simulink model "prova"  (R2023b)
settings: Solver=ode4  StartTime=0.0  StopTime=tf  FixedStep=t_step  RelTol=1e-3
values from neighbouring files (symbols this model uses):
  ARW = ARW*[1 1 1]'    [gyroscope.m]
  bias = bias*[1 1 1]'    [gyroscope.m]
  I = [Ix 0 0; 0 Iy 0; 0 0 Iz]    [gyroscope.m]
  I_inv = inv(I)    [gyroscope.m]
undefined symbols (not defined in the file or in its folder): A_1, A_2, A_3, A_4, A_5, A_6, alpha, DCM_eci_per, e, FS, H0, h_r_0, i, I_RW, I_vector_RW, inc_tot, InitialTrueAnomalyOfEarth, j_b, matrix_RW_config, matrix_RW_config_inv, mu_E, N_1, N_2, N_3, N_4, N_5, N_6, n_e, p, q0, r_1, r_2, r_3, r_4, r_5, r_6, R_E, rho_d1, rho_d2, rho_d3, rho_d4, rho_d5, rho_d6, rho_s1, rho_s2, rho_s3, rho_s4, rho_s5, rho_s6, t_step, th0, ts_sensor, w0, w0_RW, w_E, wMax_RW
libraries: matrix_library x28, simulink x4, dspindex x3, vrlib x2, aerolibutil x1
(part 1 of 2)
settings Model: Creator=samue  LastModifiedBy=samue

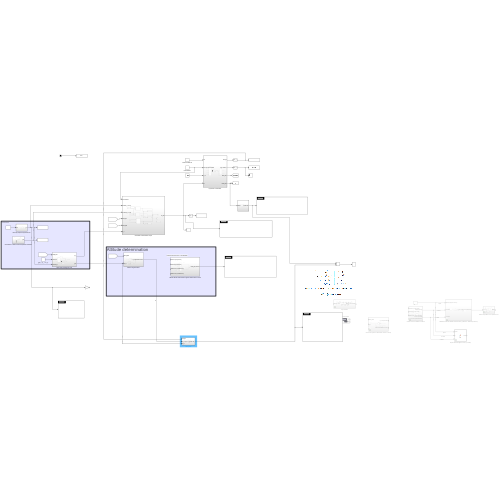
[thumbnail: Simulink's stored preview of the top-level diagram]
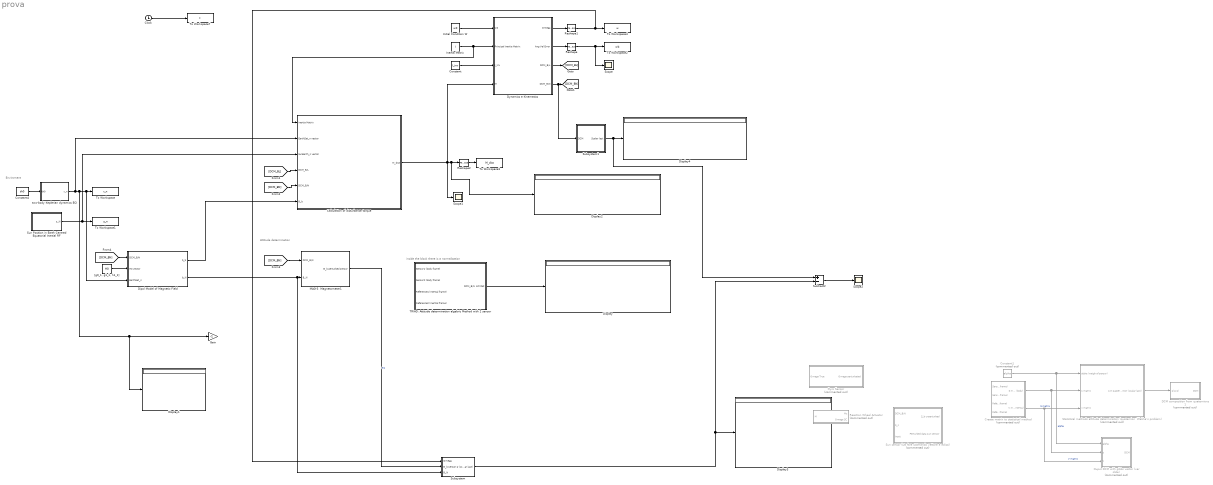
== system prova ==
  note: Attitude determination
  note: inside the block there is a normalisation
  note: Enviroment
  Calculation of disturbance torque : Subsystem
  Clock : Clock
  Constant : Constant  Value=I_inv
  Constant1 : Constant  Commented=on  Value=alpha
  Constant4 : Constant  Value=th0
  Create matrix to statistical method : Subsystem  Commented=on
  DCM composition from quaternions 1 : Subsystem  Commented=on  AncestorBlock=LibrarySAD5/DCM composition from quaternions
  Dipol Model of Magnetic Field : Subsystem
  Display{,1..4} (5 alike) : Display
  Dynamics e Kinematics : Subsystem
  Gain : Gain  Gain=-1
  Gyro Sensor : Subsystem  Commented=on
  Inertia Matrix : Constant  Value=I  VectorParams1D=off
  Initial Condition W : Constant  Value=w0
  MAG-3  Magnetometer1 : Subsystem
  Ouput DCM with gibbs vector (ver slide) : MATLAB Function  Commented=on  TreatAsAtomicUnit=on
  Reaction Wheel Actuator : Subsystem  Commented=on
  Reshape : Reshape
  Reshape1 : Reshape
  Reshape2 : Reshape
  Scope : Scope
  Scope1 : Scope
  Scope2 : Scope
  "Statistical methods attitude determination (quaternion  Wabha’s problem) " : Subsystem  Commented=on
  Subsystem : Subsystem
  Subsystem1 : Subsystem
  Subtract2 : Sum  Inputs=+-
  Sun Position in Earth Centred Equatorial Inertial RF : Subsystem
  Sun sensor (Da fare sistmando vettore e eclissi) : Subsystem  Commented=on
  TRIAD: Attitude determination algebric Method with 2 sensor : Subsystem
  To Workspace : ToWorkspace  VariableName=r_n  SampleTime=-1
  To Workspace1 : ToWorkspace  VariableName=s_n  SampleTime=-1
  To Workspace2 : ToWorkspace  VariableName=wb  SampleTime=-1
  To Workspace3 : ToWorkspace  VariableName=M_dist  SaveFormat=Timeseries  SampleTime=-1
  To Workspace4 : ToWorkspace  VariableName=w  SampleTime=-1
  To Workspace7 : ToWorkspace  VariableName=t  SampleTime=-1
  "[g0_1, g1_1, h1_1]" : Constant  Value=H0
  two-body Keplerian dynamics ECI : Subsystem
  wires:
  Inertia Matrix/1 -> Calculation of disturbance torque/1(Inertia Matrix), Dynamics e Kinematics/2(Principal Inertia Matrix)
  [DCM_BN] -> MAG-3  Magnetometer1/1(DCM_B/N)
  Constant4/1 -> two-body Keplerian dynamics ECI/1(th0)
  Constant/1 -> Dynamics e Kinematics/3(I_inv)
  [DCM_BL] -> Calculation of disturbance torque/4(DCM_B/L)
  Sun Position in Earth Centred Equatorial Inertial RF/1(s_N) -> To Workspace1/1, Calculation of disturbance torque/3(SunEarth_n vector)
  Reshape1/1 -> Subsystem/1(Omega), To Workspace4/1
  Dynamics e Kinematics/3(DCM_B/L) -> [DCM_BL]
  Reshape/1 -> Scope/1, To Workspace2/1
  Calculation of disturbance torque/1(M_dist) -> Display2/1, Reshape2/1, Dynamics e Kinematics/4(M), Scope1/1
  Dynamics e Kinematics/2(Ang Vel Error) -> Reshape/1
  Reshape2/1 -> To Workspace3/1
  "[g0_1, g1_1, h1_1]"/1 -> Dipol Model of Magnetic Field/2(H0 vector)
  "Statistical methods attitude determination (quaternion  Wabha’s problem) "/1(q in quaternion (scalar last)) -> DCM composition from quaternions 1/1(q(4x1))
  Dynamics e Kinematics/1(Omega) -> Reshape1/1
  Dynamics e Kinematics/4(DCM_B/N) -> Subsystem1/1(DCM), [DCM_BN]
  Clock/1 -> To Workspace7/1
  [DCM_BN] -> Dipol Model of Magnetic Field/1(DCM_B/N)
  Dipol Model of Magnetic Field/1(b_b) -> Calculation of disturbance torque/6(B_b)
  Create matrix to statistical method/2(V matrix (inertia)) -> "Statistical methods attitude determination (quaternion  Wabha’s problem) "/3(v matrix), Ouput DCM with gibbs vector (ver slide)/3(v)  "V matrix"
  Initial Condition W/1 -> Dynamics e Kinematics/1(w0)
  [DCM_BN] -> Calculation of disturbance torque/5(DCM_B/N)
  TRIAD: Attitude determination algebric Method with 2 sensor/1(DCM_B/N  Att Det) -> Display/1
  two-body Keplerian dynamics ECI/1(r_n) -> Calculation of disturbance torque/2(EarthSat_n vector), To Workspace/1, Dipol Model of Magnetic Field/3(EarthSat_n), Display1/1, Gain/1
  Create matrix to statistical method/1(S matrix (body)) -> "Statistical methods attitude determination (quaternion  Wabha’s problem) "/2(s matrix), Ouput DCM with gibbs vector (ver slide)/2(s)  "S matrix"
  Constant1/1 -> "Statistical methods attitude determination (quaternion  Wabha’s problem) "/1(alpha (weigh of sensor)), Ouput DCM with gibbs vector (ver slide)/1(alpha)  "alpha"
  Dipol Model of Magnetic Field/2(b_N) -> Subsystem/3(B_N), MAG-3  Magnetometer1/2(B_N)
  Subsystem1/1(Scalar last) -> Subtract2/1, Display4/1
  Subtract2/1 -> Scope2/1
  Subsystem/1(q (scalar last)) -> Subtract2/2, Display3/1
  MAG-3  Magnetometer1/1(B_b perturbed sensor) -> Subsystem/2(B_b sensor)  "B1"

== system prova/Calculation of disturbance torque ==
  Inertia Matrix : Inport
  EarthSat_n vector : Inport  Port=2
  SunEarth_n vector : Inport  Port=3
  DCM_B/L : Inport  Port=4
  DCM_B/N : Inport  Port=5
  B_b : Inport  Port=6
  Display : Display
  Extract Diagonal : matrix_library/Extract Diagonal
      settings: LibrarySourceBlock=|
      | simulink/Matrix
      | Operations/Extract Diagonal
  M of gravity gradient1 : Subsystem
  Magnetic Torque : Subsystem
  Reshape : Reshape
  Reshape1 : Reshape
  Scope : Scope
  Solar pressure on 6 faces : Subsystem  Commented=on
  Sum : Sum  Inputs=|+++
  Terminator : Terminator  Commented=on
  To Workspace1 : ToWorkspace  VariableName=M_b  SampleTime=-1
  To Workspace3 : ToWorkspace  VariableName=M_GG  SampleTime=-1
  To Workspace8 : ToWorkspace  VariableName=M_SRP  SampleTime=-1
  j_b : Constant  Value=j_b
  M_dist : Outport
  wires:
  DCM_B/L/1 -> M of gravity gradient1/2(A_B/L)
  j_b/1 -> Magnetic Torque/1(j_b)
  Magnetic Torque/1(M_b) -> Sum/3, Reshape1/1
  B_b/1 -> Magnetic Torque/2(B_b)
  Inertia Matrix/1 -> Extract Diagonal/1
  EarthSat_n vector/1 -> M of gravity gradient1/3(r_N), Solar pressure on 6 faces/2(S_N)
  DCM_B/N/1 -> Solar pressure on 6 faces/1(DCM)
  SunEarth_n vector/1 -> Solar pressure on 6 faces/3("r_N ")
  Sum/1 -> M_dist/1
  Reshape/1 -> To Workspace8/1
  Reshape1/1 -> To Workspace1/1
  M of gravity gradient1/1(GravityGradient_M) -> Reshape/1, To Workspace3/1, Sum/1
  Solar pressure on 6 faces/2(Ftot_SP) -> Terminator/1
  Solar pressure on 6 faces/1(Mtot_SP) -> Display/1, Scope/1, Sum/2
  Extract Diagonal/1 -> M of gravity gradient1/1(Inertia Vector)

== system prova/Create matrix to statistical method ==
  Sensor1 (body frame) : Inport
  Sensor2 (body frame) : Inport  Port=2
  Reference1 (Inertial frame) : Inport  Port=3
  Reference2 (Inertial frame) : Inport  Port=4
  Matrix Concatenate1 : Concatenate  Mode=Multidimensional array  ConcatenateDimension=2
  Matrix Concatenate2 : Concatenate  Mode=Multidimensional array  ConcatenateDimension=2
  Normalize Vector1 : Subsystem
  Normalize Vector2 : Subsystem
  Normalize Vector3 : Subsystem
  Normalize Vector4 : Subsystem
  S matrix (body) : Outport
  V matrix (inertia) : Outport  Port=2
  wires:
  Matrix Concatenate1/1 -> V matrix (inertia)/1
  Normalize Vector1/1(Versor) -> Matrix Concatenate2/1
  Normalize Vector2/1(Versor) -> Matrix Concatenate2/2
  Normalize Vector4/1(Versor) -> Matrix Concatenate1/2
  Normalize Vector3/1(Versor) -> Matrix Concatenate1/1
  Matrix Concatenate2/1 -> S matrix (body)/1
  Reference1 (Inertial frame)/1 -> Normalize Vector3/1(Vector)
  Reference2 (Inertial frame)/1 -> Normalize Vector4/1(Vector)
  Sensor1 (body frame)/1 -> Normalize Vector1/1(Vector)
  Sensor2 (body frame)/1 -> Normalize Vector2/1(Vector)

== system prova/DCM composition from quaternions 1 ==
  q(4x1) : Inport
  Cross product matrix composition : Subsystem
  Demux : Demux
  Dot Product : DotProduct  OutDataTypeStr=Inherit: Inherit via internal rule
  Gain : Gain  Gain=[1 0 0; 0 1 0; 0 0 1]
  Gain1 : Gain  Gain=2
  Gain2 : Gain  Gain=-2
  Mux : Mux  Inputs=3
  Product : Product  Multiplication=Matrix(*)
  Product1 : Product
  Square : Math  Operator=square
  Sum : Sum  Inputs=|-+
  Sum1 : Sum  Inputs=+++
  Transpose : Math  Operator=transpose
  DCM : Outport
  wires:
  Gain/1 -> Sum1/1
  Demux/1 -> Mux/1
  q(4x1)/1 -> Demux/1
  Demux/2 -> Mux/2
  Mux/1 -> Dot Product/2, Dot Product/1, Product/1, Cross product matrix composition/1(q_vect), Transpose/1  "q_vect"
  Demux/4 -> Gain2/1, Square/1  "q4"
  Demux/3 -> Mux/3
  Dot Product/1 -> Sum/1
  Sum/1 -> Gain/1
  Square/1 -> Sum/2
  Transpose/1 -> Product/2
  Product/1 -> Gain1/1
  Gain2/1 -> Product1/2
  Cross product matrix composition/1(q_vect cross) -> Product1/1  "omega_mat"
  Product1/1 -> Sum1/3
  Gain1/1 -> Sum1/2
  Sum1/1 -> DCM/1

== system prova/Dipol Model of Magnetic Field ==
  note: CODE TO ADD
      | % Definition of Magnetic Field (Dipole model)
      |  j_b = [0.01 0.05 0.01]';
      | H0 = 1e-9.*[-29404.8 -1450.9 4652.5]';
  DCM_B/N : Inport
  H0 vector : Inport  Port=2
  EarthSat_n : Inport  Port=3
  Calculation of b_n : Subsystem
  Matrix Multiply : Product  Multiplication=Matrix(*)
  To Workspace : ToWorkspace  VariableName=bn  SampleTime=-1
  b_b : Outport
  b_N : Outport  Port=2
  wires:
  Matrix Multiply/1 -> b_b/1
  DCM_B/N/1 -> Matrix Multiply/1
  H0 vector/1 -> Calculation of b_n/1(H0 vector)
  EarthSat_n/1 -> Calculation of b_n/2(EarthSat_n)
  Calculation of b_n/1(b_N) -> Matrix Multiply/2, To Workspace/1, b_N/1

== system prova/Dynamics e Kinematics ==
  w0 : Inport
  Principal Inertia Matrix : Inport  Port=2
  I_inv : Inport  Port=3
  M : Inport  Port=4
  Attitude error GG : Subsystem
  Constant6 : Constant  Value=q0
  DCM composition from quaternions 1 : Subsystem  AncestorBlock=LibrarySAD5/DCM composition from quaternions
  Kinematics quaternion2 : Subsystem
  Single spin dynamics : Subsystem  AncestorBlock=My_library/Single spin dynamics
  Terminator1 : Terminator
  Omega : Outport
  Ang Vel Error : Outport  Port=2
  DCM_B/L : Outport  Port=3
  DCM_B/N : Outport  Port=4
  wires:
  DCM composition from quaternions 1/1(DCM) -> DCM_B/N/1, Attitude error GG/2(DCM_B/N)
  Constant6/1 -> Kinematics quaternion2/2(q0)
  Single spin dynamics/1(Omega) -> Omega/1, Attitude error GG/1(w), Kinematics quaternion2/1(omega)
  Kinematics quaternion2/2(q^(-1)) -> Terminator1/1
  M/1 -> Single spin dynamics/4(M)
  w0/1 -> Single spin dynamics/3(Omega_0)
  Principal Inertia Matrix/1 -> Single spin dynamics/2(Inertia matrix)
  Kinematics quaternion2/1(q) -> DCM composition from quaternions 1/1(q(4x1))
  Attitude error GG/2(DCM_B/L) -> DCM_B/L/1
  Attitude error GG/1(Ang Vel Error) -> Ang Vel Error/1
  I_inv/1 -> Single spin dynamics/1(Inertia matrix inverse)

== system prova/Gyro Sensor ==
  Omega True : Inport
  Band-Limited White Noise : simulink/Sources/Band-Limited White Noise  Cov=[0.00001]  Ts=0.1  seed=[23341]
  Constant : Constant  Value=ARW  VectorParams1D=off
  Constant1 : Constant  Value=bias  VectorParams1D=off
  Sum : Sum  Inputs=|++
  Sum1 : Sum  Inputs=|++
  Sum2 : Sum  Inputs=|++
  Zero-Order Hold : ZeroOrderHold  SampleTime=-1
  Omega perturbated : Outport
  wires:
  Zero-Order Hold/1 -> Sum/1
  Sum2/1 -> Omega perturbated/1
  Sum1/1 -> Sum2/1
  Sum/1 -> Sum1/1
  Omega True/1 -> Zero-Order Hold/1
  Constant1/1 -> Sum2/2
  Band-Limited White Noise/1 -> Sum/2
  Constant/1 -> Sum1/2

== system prova/MAG-3  Magnetometer1 ==
  note: CODE TO ADD TO MAKE SENSOR WORK
      | % Time definition
      | t0 = 0;
      | tf = T; %Period of orbit
      | t_step = 0.01; %fixed step of simulation
      | ts_sensor = t_step; % Sample of sensor (can change but must to be a multiple of t_step)
      |
      | % MAG-3 sensor data and error
      | FS = 500e-9; %Full scale value
      | inc_lin = 0.15/100; % Accuracy error
      | inc_acc = 0.75/100; % Linear error
      | inc_tot = sqrt(inc_lin^2 + inc_acc^2); %Total error
  DCM_B/N : Inport
  B_N : Inport  Port=2
  Error gain of sensor MAG-3 : Gain  Gain=inc_tot*FS
  Rotation in body frame : Product  Multiplication=Matrix(*)
  Saturation to FS : Saturate  UpperLimit=FS  LowerLimit=-FS
  Sum : Sum  Inputs=|++
  Vector Concatenate : Concatenate  NumInputs=3
  White Noise : RandomNumber  DisableCoverage=on  Seed=1  SampleTime=ts_sensor
  White Noise1 : RandomNumber  DisableCoverage=on  Seed=2  SampleTime=ts_sensor
  White Noise2 : RandomNumber  DisableCoverage=on  Seed=3  SampleTime=ts_sensor
  Zero-Order Hold : ZeroOrderHold  SampleTime=ts_sensor
  B_b perturbed sensor : Outport
  wires:
  Vector Concatenate/1 -> Error gain of sensor MAG-3/1
  White Noise/1 -> Vector Concatenate/1
  Error gain of sensor MAG-3/1 -> Sum/2
  White Noise2/1 -> Vector Concatenate/3
  White Noise1/1 -> Vector Concatenate/2
  DCM_B/N/1 -> Rotation in body frame/1
  B_N/1 -> Zero-Order Hold/1
  Zero-Order Hold/1 -> Rotation in body frame/2
  Saturation to FS/1 -> B_b perturbed sensor/1
  Rotation in body frame/1 -> Sum/1
  Sum/1 -> Saturation to FS/1

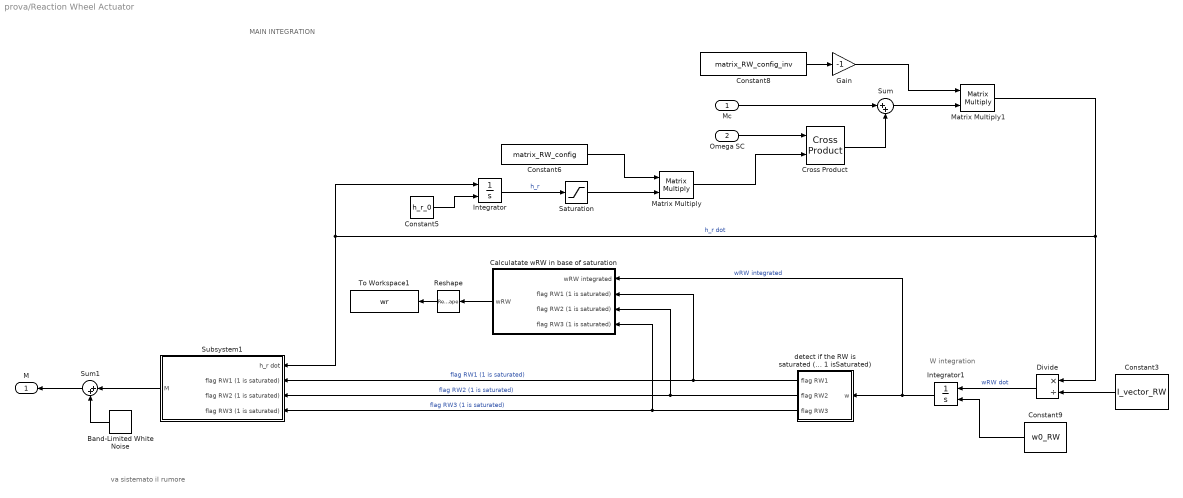
== system prova/Reaction Wheel Actuator ==
  note: W integration
  note: va sistemato il rumore
  note: MAIN INTEGRATION
  Mc : Inport
  Omega SC : Inport  Port=2
  Band-Limited White Noise : simulink/Sources/Band-Limited White Noise  Cov=[0.00001]  Ts=t_step  seed=[23341]
  Calculatate wRW in base of saturation : Subsystem
  Constant3 : Constant  Value=I_vector_RW
  Constant5 : Constant  Value=h_r_0  VectorParams1D=off
  Constant6 : Constant  Value=matrix_RW_config  VectorParams1D=off
  Constant8 : Constant  Value=matrix_RW_config_inv  VectorParams1D=off
  Constant9 : Constant  Value=w0_RW
  Cross Product : matrix_library/Cross Product
  Divide : Product  Inputs=*/
  Gain : Gain  Gain=-1
  Integrator : Integrator  InitialConditionSource=external
  Integrator1 : Integrator  InitialConditionSource=external
  Matrix Multiply : Product  Multiplication=Matrix(*)
  Matrix Multiply1 : Product  Multiplication=Matrix(*)
  Reshape : Reshape
  Saturation : Saturate  UpperLimit=wMax_RW*I_RW  LowerLimit=-wMax_RW*I_RW
  Subsystem1 : Subsystem
  Sum : Sum  Inputs=|++
  Sum1 : Sum  Inputs=|++
  To Workspace1 : ToWorkspace  VariableName=wr  SampleTime=-1
  detect if the RW is saturated (output == 1 isSaturated) : Subsystem
  M : Outport
  wires:
  Matrix Multiply1/1 -> Integrator/1, Subsystem1/1(h_r dot), Divide/1  "h_r dot"
  Constant6/1 -> Matrix Multiply/1
  Cross Product/1 -> Sum/2
  Constant8/1 -> Gain/1
  Sum/1 -> Matrix Multiply1/2
  detect if the RW is saturated (output == 1 isSaturated)/2(flag RW2) -> Calculatate wRW in base of saturation/3(flag RW2 (1 is saturated)), Subsystem1/3(flag RW2 (1 is saturated))  "flag RW2 (1 is saturated)"
  Calculatate wRW in base of saturation/1(wRW) -> Reshape/1
  Matrix Multiply/1 -> Cross Product/2
  Constant5/1 -> Integrator/2
  Constant3/1 -> Divide/2
  Gain/1 -> Matrix Multiply1/1
  Mc/1 -> Sum/1
  Saturation/1 -> Matrix Multiply/2
  Integrator1/1 -> Calculatate wRW in base of saturation/1(wRW integrated), detect if the RW is saturated (output == 1 isSaturated)/1(w)  "wRW integrated"
  Constant9/1 -> Integrator1/2
  Divide/1 -> Integrator1/1  "wRW dot"
  Integrator/1 -> Saturation/1  "h_r"
  detect if the RW is saturated (output == 1 isSaturated)/3(flag RW3) -> Calculatate wRW in base of saturation/4(flag RW3 (1 is saturated)), Subsystem1/4(flag RW3 (1 is saturated))  "flag RW3 (1 is saturated)"
  detect if the RW is saturated (output == 1 isSaturated)/1(flag RW1) -> Calculatate wRW in base of saturation/2(flag RW1 (1 is saturated)), Subsystem1/2(flag RW1 (1 is saturated))  "flag RW1 (1 is saturated)"
  Reshape/1 -> To Workspace1/1
  Omega SC/1 -> Cross Product/1
  Subsystem1/1(M) -> Sum1/1
  Sum1/1 -> M/1
  Band-Limited White Noise/1 -> Sum1/2

== system prova/Statistical methods attitude determination (quaternion  Wabha’s problem)  ==
  note: In questo blocco ci sono altri metodi per il calcolo di q
  note: BLOCCO DA SISTEMARE SCEGLIENDO UNA SOLUZIONE
  note: Resolve linear system:
      | (𝑆 − σI)𝑞 + zq_4 = 𝜆_(MAX)*𝑞
      | 𝑧'𝑞 + σ*q_4 = 𝜆_(MAX)*𝑞_4
      |
      | Calculate eigenvalue (in the theory we assumed that lambda_max = 1)
  note: 𝐾 = [ (𝑆 − σI), 𝑧
      | 𝑧 ' 𝜎 ]
  note: 𝑧 = [𝑏23 − 𝑏32 , b31 − 𝑏13 , b12 − 𝑏21] '
  alpha (weigh of sensor) : Inport
  s matrix : Inport  Port=2
  v matrix : Inport  Port=3
  Adjoint of 3x3 Matrix : aerolibutil/Adjoint of 3x3 Matrix
  Blocco da convertire in formato simulink. Ho trovato 3 soluzioni differenti al proble : MATLAB Function  TreatAsAtomicUnit=on
  For Iterator Subsystem to calculate B matrix : Subsystem  TreatAsAtomicUnit=on
  Gain : Gain  Gain=eye(3)
  Matrix Concatenate : Concatenate  Mode=Multidimensional array  ConcatenateDimension=2
  Matrix Concatenate1 : Concatenate  Mode=Multidimensional array
  Matrix trace : Subsystem
  Subtract : Sum  Inputs=+-
  Sum : Sum  Inputs=|++
  Transpose : Math  Operator=transpose
  Transpose2 : Math  Operator=transpose
  Vector Concatenate1 : Concatenate
  Vector z : Subsystem
  q in quaternion (scalar last) : Outport
  wires:
  Transpose/1 -> Sum/2
  For Iterator Subsystem to calculate B matrix/1(B matrix) -> Vector z/1(B), Matrix trace/1(Matrix), Transpose/1, Sum/1  "B matrix"
  Sum/1 -> Adjoint of 3x3 Matrix/1, Blocco da convertire in formato simulink. Ho trovato 3 soluzioni differenti al proble/2(S), Subtract/1  "matrix S"
  Gain/1 -> Subtract/2
  Matrix trace/1(trace) -> Vector Concatenate1/2, Gain/1  "sigma = tr(B)"
  Matrix Concatenate/1 -> Matrix Concatenate1/1
  Vector Concatenate1/1 -> Transpose2/1
  Vector z/1(z) -> Vector Concatenate1/1, Matrix Concatenate/2
  Transpose2/1 -> Matrix Concatenate1/2
  Subtract/1 -> Matrix Concatenate/1  "S - sigma*eye(3)"
  alpha (weigh of sensor)/1 -> For Iterator Subsystem to calculate B matrix/1(alpha)
  v matrix/1 -> For Iterator Subsystem to calculate B matrix/3(v matrix)
  s matrix/1 -> For Iterator Subsystem to calculate B matrix/2(s matrix)
  Blocco da convertire in formato simulink. Ho trovato 3 soluzioni differenti al proble/1(q) -> q in quaternion (scalar last)/1  "q in quaternion (scalar last)"
  Adjoint of 3x3 Matrix/1 -> Blocco da convertire in formato simulink. Ho trovato 3 soluzioni differenti al proble/3(Sadj)
  Matrix Concatenate1/1 -> Blocco da convertire in formato simulink. Ho trovato 3 soluzioni differenti al proble/1(K)  "K matrix"

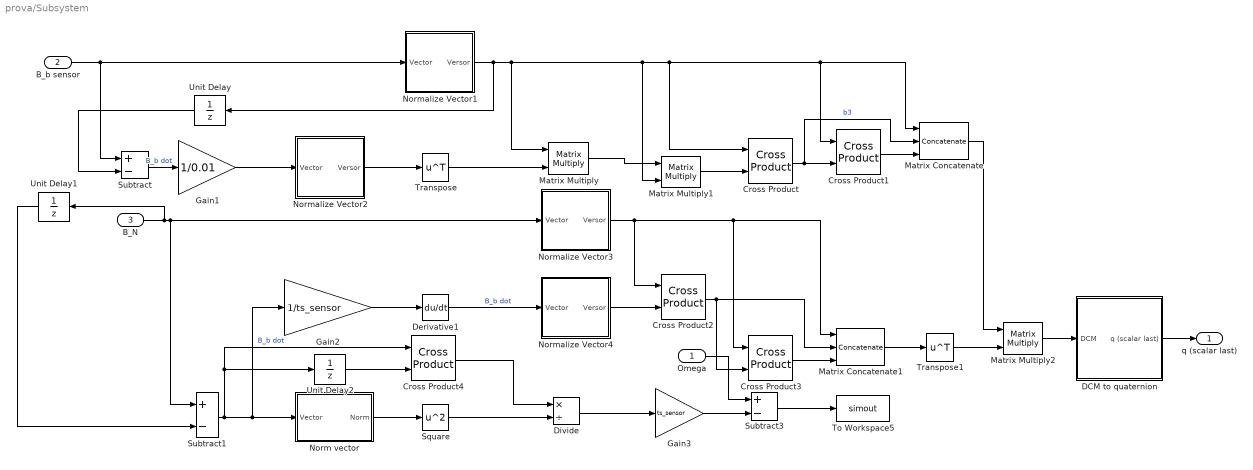
== system prova/Subsystem ==
  Omega : Inport
  B_b sensor : Inport  Port=2
  B_N : Inport  Port=3
  Cross Product{,1..4} (5 alike) : matrix_library/Cross Product
  DCM to quaternion : Subsystem
  Derivative1 : Derivative
  Divide : Product  Inputs=*/
  Gain1 : Gain  Gain=1/0.01
  Gain2 : Gain  Gain=1/ts_sensor
  Gain3 : Gain  Gain=ts_sensor
  Matrix Concatenate : Concatenate  NumInputs=3  Mode=Multidimensional array  ConcatenateDimension=2
  Matrix Concatenate1 : Concatenate  NumInputs=3  Mode=Multidimensional array  ConcatenateDimension=2
  Matrix Multiply : Product  Multiplication=Matrix(*)
  Matrix Multiply1 : Product  Multiplication=Matrix(*)
  Matrix Multiply2 : Product  Multiplication=Matrix(*)
  Norm vector : Subsystem  AncestorBlock=LibrarySAD5/Normalize Vector1
  Normalize Vector1 : Subsystem
  Normalize Vector2 : Subsystem
  Normalize Vector3 : Subsystem
  Normalize Vector4 : Subsystem
  Square : Math  Operator=square
  Subtract : Sum  Inputs=+-
  Subtract1 : Sum  Inputs=+-
  Subtract3 : Sum  Inputs=+-
  To Workspace5 : ToWorkspace  VariableName=simout  SaveFormat=Timeseries  SampleTime=-1
  Transpose : Math  Operator=transpose
  Transpose1 : Math  Operator=transpose
  Unit Delay : UnitDelay  SampleTime=-1  HasFrameUpgradeWarning=on
  Unit Delay1 : UnitDelay  SampleTime=-1  HasFrameUpgradeWarning=on
  Unit Delay2 : UnitDelay  SampleTime=-1  HasFrameUpgradeWarning=on
  q (scalar last) : Outport
  wires:
  Unit Delay1/1 -> Subtract1/2
  B_b sensor/1 -> Normalize Vector1/1(Vector), Subtract/1
  Gain1/1 -> Normalize Vector2/1(Vector)
  Subtract/1 -> Gain1/1  "B_b dot"
  Unit Delay/1 -> Subtract/2
  B_N/1 -> Normalize Vector3/1(Vector), Subtract1/1, Unit Delay1/1
  Subtract1/1 -> Norm vector/1(Vector), Gain2/1, Cross Product4/1, Unit Delay2/1  "B_b dot"
  Normalize Vector2/1(Versor) -> Transpose/1
  Gain2/1 -> Derivative1/1
  Unit Delay2/1 -> Cross Product4/2
  Norm vector/1(Norm) -> Square/1
  Normalize Vector1/1(Versor) -> Cross Product1/1, Matrix Concatenate/1, Cross Product/1, Matrix Multiply1/2, Matrix Multiply/1, Unit Delay/1
  Transpose/1 -> Matrix Multiply/2
  Derivative1/1 -> Normalize Vector4/1(Vector)  "B_b dot"
  Cross Product4/1 -> Divide/1
  Square/1 -> Divide/2
  Matrix Multiply/1 -> Matrix Multiply1/1
  Normalize Vector3/1(Versor) -> Matrix Concatenate1/1, Cross Product3/1, Cross Product2/1
  Normalize Vector4/1(Versor) -> Cross Product2/2
  Divide/1 -> Gain3/1
  Matrix Multiply1/1 -> Cross Product/2
  Cross Product2/1 -> Matrix Concatenate1/2, Cross Product3/2
  Omega/1 -> Subtract3/1
  Gain3/1 -> Subtract3/2
  Cross Product/1 -> Cross Product1/2, Matrix Concatenate/2  "b3"
  Cross Product3/1 -> Matrix Concatenate1/3
  Subtract3/1 -> To Workspace5/1
  Cross Product1/1 -> Matrix Concatenate/3
  Matrix Concatenate1/1 -> Transpose1/1
  Matrix Concatenate/1 -> Matrix Multiply2/1
  Transpose1/1 -> Matrix Multiply2/2
  Matrix Multiply2/1 -> DCM to quaternion/1(DCM)
  DCM to quaternion/1(q (scalar last)) -> q (scalar last)/1

== system prova/Subsystem1 ==
  DCM : Inport
  Constant : Constant
  Divide : Product  Inputs=*/
  Extract Diagonal : matrix_library/Extract Diagonal
      settings: LibrarySourceBlock=|
      | simulink/Matrix
      | Operations/Extract Diagonal
  Gain : Gain  Gain=0.5
  Gain1 : Gain  Gain=[0 0 0; 0 0 1; 0 -1 0]
  Gain2 : Gain  Gain=[0 0 -1; 0 0 0; 1 0 0]
  Gain3 : Gain  Gain=[0 1 0; -1 0 0; 0 0 0]
  Gain4 : Gain  Gain=4
  Normalize Vector1 : Subsystem
  Sqrt : Sqrt
  Sum : Sum  Inputs=|++
  Sum of Elements{,1..3} (4 alike) : Sum  Inputs=+
  Vector Concatenate : Concatenate  NumInputs=3
  Vector Concatenate1 : Concatenate
  Scalar last : Outport
  wires:
  Extract Diagonal/1 -> Sum of Elements/1
  Sum of Elements/1 -> Sum/1
  Constant/1 -> Sum/2
  Sum/1 -> Sqrt/1
  Sqrt/1 -> Gain/1
  DCM/1 -> Gain1/1, Gain2/1, Gain3/1, Extract Diagonal/1
  Gain2/1 -> Sum of Elements1/1
  Sum of Elements1/1 -> Vector Concatenate/2
  Gain1/1 -> Sum of Elements2/1
  Sum of Elements2/1 -> Vector Concatenate/1
  Sum of Elements3/1 -> Vector Concatenate/3
  Gain3/1 -> Sum of Elements3/1
  Vector Concatenate/1 -> Divide/1
  Gain/1 -> Vector Concatenate1/2, Gain4/1
  Gain4/1 -> Divide/2
  Divide/1 -> Vector Concatenate1/1
  Vector Concatenate1/1 -> Normalize Vector1/1(Vector)
  Normalize Vector1/1(Versor) -> Scalar last/1

== system prova/Sun Position in Earth Centred Equatorial Inertial RF ==
  note: pointing Sun from Earth
      |
      | x=vernal line
      | y=perpendicular
      | z=cnp
  Clock : Clock
  Gain : Gain  Gain=cos(23.45/360*2*pi)
  Gain1 : Gain  Gain=sin(23.45/360*2*pi)
  InitialTrueAnomalyOfEarth : Constant  Value=InitialTrueAnomalyOfEarth
  MatrixMultiply : Product
  Mux : Mux  Inputs=3
  Product : Product
  Sum : Sum  Inputs=|++
  Trigonometric Function : Trigonometry  Operator=cos
  Trigonometric Function1 : Trigonometry
  mean ang vel : Constant  Value=2*pi/31536000
  mean distance : Constant  Value=149597870
  s_N : Outport
  wires:
  Trigonometric Function/1 -> Mux/1
  Gain1/1 -> Mux/3
  Mux/1 -> MatrixMultiply/2
  MatrixMultiply/1 -> s_N/1  "s_N"
  mean distance/1 -> MatrixMultiply/1
  Gain/1 -> Mux/2
  Trigonometric Function1/1 -> Gain1/1, Gain/1
  mean ang vel/1 -> Product/2
  Clock/1 -> Product/1
  InitialTrueAnomalyOfEarth/1 -> Sum/2
  Product/1 -> Sum/1
  Sum/1 -> Trigonometric Function1/1, Trigonometric Function/1

== system prova/Sun sensor (Da fare sistmando vettore e eclissi) ==
  note: SUN SENSOR DA RIFINIRE, ma Utilizzabile
      | -> Modellare non rilevamento sole (esempio eclissi)
      | -> Modellare albedo terra/luna per riflessi
      | -> Sistemare distrubi basandosi su sensore reale
  DCM_B/N : Inport
  S_n : Inport  Port=2
  Input : Inport  Port=3
  Band-Limited White Noise : simulink/Sources/Band-Limited White Noise  Cov=5e9*[1 1 1]  Ts=ts_sensor  seed=[23341]
  Normalize Vector1 : Subsystem
  Rotation in body frame : Product  Multiplication=Matrix(*)
  Rotation in body frame1 : Product  Multiplication=Matrix(*)
  Sum : Sum  Inputs=|++
  Zero-Order Hold : ZeroOrderHold  SampleTime=ts_sensor
  S_b unperturbed : Outport
  Perturbed data sun sensor : Outport  Port=2
  wires:
  Band-Limited White Noise/1 -> Sum/2
  DCM_B/N/1 -> Rotation in body frame/1, Rotation in body frame1/1
  S_n/1 -> Zero-Order Hold/1, Normalize Vector1/1(Vector)
  Normalize Vector1/1(Versor) -> Rotation in body frame/2
  Zero-Order Hold/1 -> Rotation in body frame1/2
  Rotation in body frame1/1 -> Sum/1
  Rotation in body frame/1 -> S_b unperturbed/1
  Sum/1 -> Perturbed data sun sensor/1

== system prova/TRIAD: Attitude determination algebric Method with 2 sensor ==
  note: 𝑉^(-1) = 𝑉';
      | 𝐴 = 𝑆𝑉^(-1) = 𝑆𝑉'
  note: 𝑣1 = 𝑎;
      | 𝑣2 = (𝑎 ∧ 𝑏)/|𝑎 ∧ 𝑏|;
      | 𝑣3 = 𝑎 ∧ 𝑣2
  note: S1 = 𝑝;
      | 𝑠2 = (𝑝 ∧ 𝑞)/(|𝑝 ∧ 𝑞|);
      | 𝑠3 = 𝑝 ∧ 𝑠2
  Sensor1 (body frame) : Inport
  Sensor2 (body frame) : Inport  Port=2
  Reference1 (Inertial frame) : Inport  Port=3
  Reference2 (Inertial frame) : Inport  Port=4
  Matrix Multiply : Product  Multiplication=Matrix(*)
  Normalize Vector1 : Subsystem
  Normalize Vector2 : Subsystem
  Normalize Vector3 : Subsystem
  Normalize Vector4 : Subsystem
  Subsystem : Subsystem
  Subsystem1 : Subsystem
  Transpose : Math  Operator=transpose
  DCM_B/N  Att Det : Outport
  wires:
  Sensor1 (body frame)/1 -> Normalize Vector2/1(Vector)  "q"
  Sensor2 (body frame)/1 -> Normalize Vector3/1(Vector)  "p"
  Subsystem/1("Matrix S Measurements ") -> Matrix Multiply/1  "Matrix S Measurements (body frame)"
  Normalize Vector2/1(Versor) -> Subsystem/1(versor p (body frame))
  Normalize Vector3/1(Versor) -> Subsystem/2(versor q (body frame))
  Normalize Vector1/1(Versor) -> Subsystem1/1(versor a (body frame))
  Reference2 (Inertial frame)/1 -> Normalize Vector4/1(Vector)  "b"
  Reference1 (Inertial frame)/1 -> Normalize Vector1/1(Vector)  "a"
  Subsystem1/1("Matrix V certain model ") -> Transpose/1  "Matrix V (inertial frame)"
  Normalize Vector4/1(Versor) -> Subsystem1/2(versor b (body frame))
  Matrix Multiply/1 -> DCM_B/N  Att Det/1  "DCM_B/N from attirude determination"
  Transpose/1 -> Matrix Multiply/2

== system prova/two-body Keplerian dynamics ECI ==
  th0 : Inport
  Constant : Constant  Value=DCM_eci_per
  Integretion of true anomaly : Subsystem
  Matrix Multiply : Product  Multiplication=Matrix(*)
  Transpose : Math  Operator=transpose
  r_perifocal : Subsystem
  r_n : Outport
  wires:
  th0/1 -> Integretion of true anomaly/1(th0)
  Integretion of true anomaly/1(th) -> r_perifocal/1(th)
  Constant/1 -> Transpose/1
  Transpose/1 -> Matrix Multiply/1
  r_perifocal/1(r_per) -> Matrix Multiply/2
  Matrix Multiply/1 -> r_n/1

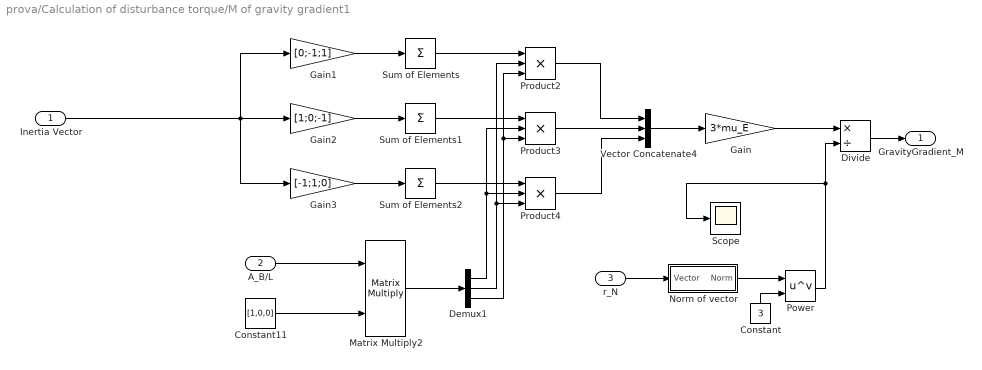
== system prova/Calculation of disturbance torque/M of gravity gradient1 ==
  Inertia Vector : Inport
  A_B/L : Inport  Port=2
  r_N : Inport  Port=3
  Constant : Constant  Value=3
  Constant11 : Constant  Value=[1,0,0]
  Demux1 : Demux  Outputs=3
  Divide : Product  Inputs=*/
  Gain : Gain  Gain=3*mu_E
  Gain1 : Gain  Gain=[0;-1;1]
  Gain2 : Gain  Gain=[1;0;-1]
  Gain3 : Gain  Gain=[-1;1;0]
  Matrix Multiply2 : Product  Multiplication=Matrix(*)
  Norm of vector : Subsystem  AncestorBlock=LibrarySAD5/Normalize Vector1
  Power : Math  Operator=pow
  Product2 : Product  Inputs=3
  Product3 : Product  Inputs=3
  Product4 : Product  Inputs=3
  Scope : Scope
  Sum of Elements : Sum  Inputs=+
  Sum of Elements1 : Sum  Inputs=+
  Sum of Elements2 : Sum  Inputs=+
  Vector Concatenate4 : Concatenate  NumInputs=3
  GravityGradient_M : Outport
  wires:
  Demux1/3 -> Product2/3, Product3/3
  Product2/1 -> Vector Concatenate4/1
  Matrix Multiply2/1 -> Demux1/1
  Product4/1 -> Vector Concatenate4/3
  Product3/1 -> Vector Concatenate4/2
  Demux1/1 -> Product4/2, Product3/2
  Constant11/1 -> Matrix Multiply2/2
  Demux1/2 -> Product4/3, Product2/2
  A_B/L/1 -> Matrix Multiply2/1
  Vector Concatenate4/1 -> Gain/1
  Gain1/1 -> Sum of Elements/1
  Gain2/1 -> Sum of Elements1/1
  Gain3/1 -> Sum of Elements2/1
  Sum of Elements/1 -> Product2/1
  Sum of Elements1/1 -> Product3/1
  Sum of Elements2/1 -> Product4/1
  Inertia Vector/1 -> Gain1/1, Gain2/1, Gain3/1
  Gain/1 -> Divide/1
  Power/1 -> Scope/1, Divide/2
  Constant/1 -> Power/2
  r_N/1 -> Norm of vector/1(Vector)
  Divide/1 -> GravityGradient_M/1
  Norm of vector/1(Norm) -> Power/1

== system prova/Calculation of disturbance torque/Magnetic Torque ==
  j_b : Inport
  B_b : Inport  Port=2
  Cross Product : matrix_library/Cross Product
  M_b : Outport
  wires:
  Cross Product/1 -> M_b/1
  j_b/1 -> Cross Product/1
  B_b/1 -> Cross Product/2

== system prova/Calculation of disturbance torque/Solar pressure on 6 faces ==
  DCM : Inport
  S_N : Inport  Port=2
  "r_N " : Inport  Port=3
  Acos : Trigonometry  Operator=acos
  Dot Product : DotProduct  OutDataTypeStr=Inherit: Inherit via internal rule
  MatrixMultiply : Product  Multiplication=Matrix(*)
  MatrixMultiply1 : Product  Multiplication=Matrix(*)
  Norm of vector : Subsystem  AncestorBlock=LibrarySAD5/Normalize Vector1
  Normalize Vector : vrlib/Utilities/Normalize Vector  maxzero=0
  Normalize Vector1 : vrlib/Utilities/Normalize Vector  maxzero=0
  Solar pressure on 6 faces1 : Subsystem
  Sum1 : Sum  Inputs=|+-
  Mtot_SP : Outport
  Ftot_SP : Outport  Port=2
  wires:
  DCM/1 -> MatrixMultiply1/1, MatrixMultiply/1
  S_N/1 -> Norm of vector/1(Vector), Sum1/1, MatrixMultiply/2, Normalize Vector1/1
  "r_N "/1 -> Sum1/2, MatrixMultiply1/2
  MatrixMultiply1/1 -> Solar pressure on 6 faces1/2(r_B)
  Norm of vector/1(Norm) -> Solar pressure on 6 faces1/5(s_N norm)
  MatrixMultiply/1 -> Solar pressure on 6 faces1/1(s_B)
  Sum1/1 -> Solar pressure on 6 faces1/4(S_N - r_N), Normalize Vector/1
  Normalize Vector/1 -> Dot Product/1
  Normalize Vector1/1 -> Dot Product/2
  Solar pressure on 6 faces1/1(Ftot_SP) -> Ftot_SP/1
  Dot Product/1 -> Acos/1
  Acos/1 -> Solar pressure on 6 faces1/3(S/E_S/sc_angle)
  Solar pressure on 6 faces1/2(Mtot_SP) -> Mtot_SP/1

== system prova/Create matrix to statistical method/Normalize Vector1 ==
  Vector : Inport
  Divide : Product  Inputs=*/
  Normalize Vector : Subsystem  AncestorBlock=LibrarySAD5/Normalize Vector1
  Versor : Outport
  wires:
  Vector/1 -> Normalize Vector/1(Vector), Divide/1
  Divide/1 -> Versor/1
  Normalize Vector/1(Norm) -> Divide/2

== system prova/Create matrix to statistical method/Normalize Vector2 ==
  Vector : Inport
  Divide : Product  Inputs=*/
  Normalize Vector : Subsystem  AncestorBlock=LibrarySAD5/Normalize Vector1
  Versor : Outport
  wires:
  Vector/1 -> Normalize Vector/1(Vector), Divide/1
  Divide/1 -> Versor/1
  Normalize Vector/1(Norm) -> Divide/2

== system prova/Create matrix to statistical method/Normalize Vector3 ==
  Vector : Inport
  Divide : Product  Inputs=*/
  Normalize Vector : Subsystem  AncestorBlock=LibrarySAD5/Normalize Vector1
  Versor : Outport
  wires:
  Vector/1 -> Normalize Vector/1(Vector), Divide/1
  Divide/1 -> Versor/1
  Normalize Vector/1(Norm) -> Divide/2

== system prova/Create matrix to statistical method/Normalize Vector4 ==
  Vector : Inport
  Divide : Product  Inputs=*/
  Normalize Vector : Subsystem  AncestorBlock=LibrarySAD5/Normalize Vector1
  Versor : Outport
  wires:
  Vector/1 -> Normalize Vector/1(Vector), Divide/1
  Divide/1 -> Versor/1
  Normalize Vector/1(Norm) -> Divide/2

== system prova/DCM composition from quaternions 1/Cross product matrix composition ==
  q_vect : Inport
  Demux : Demux  Outputs=3
  Gain : Gain  Gain=[0 0 0; 0 0 -1; 0 1 0]
  Gain1 : Gain  Gain=[0 0 1; 0 0 0; -1 0 0]
  Gain2 : Gain  Gain=[0 -1 0; 1 0 0; 0 0 0]
  Sum : Sum  Inputs=+++
  q_vect cross : Outport
  wires:
  Gain1/1 -> Sum/2
  Demux/3 -> Gain2/1
  Demux/1 -> Gain/1
  q_vect/1 -> Demux/1
  Gain2/1 -> Sum/3
  Demux/2 -> Gain1/1
  Gain/1 -> Sum/1
  Sum/1 -> q_vect cross/1

== system prova/Dipol Model of Magnetic Field/Calculation of b_n ==
  H0 vector : Inport
  EarthSat_n : Inport  Port=2
  Constant : Constant  Value=3
  Divide : Product  Inputs=*/
  Dot Product : DotProduct  OutDataTypeStr=Inherit: Inherit via internal rule
  Gain : Gain  Gain=3
  Gain1 : Gain  Gain=R_E^3
  Norm of Vector : Subsystem  AncestorBlock=LibrarySAD5/Normalize Vector1
  Norm of Vector H : Subsystem  AncestorBlock=LibrarySAD5/Normalize Vector1
  Normalize Vector : Subsystem
  Power : Math  Operator=pow
  Product : Product
  Product1 : Product
  Subtract : Sum  Inputs=+-
  m_versor : Subsystem
  b_N : Outport
  wires:
  Norm of Vector/1(Norm) -> Power/1
  Product/1 -> Subtract/1
  Divide/1 -> Gain1/1
  EarthSat_n/1 -> Norm of Vector/1(Vector), Normalize Vector/1(Vector)
  Normalize Vector/1(Versor) -> Product/1, Dot Product/1
  Gain1/1 -> Product1/1
  m_versor/1(m_versor) -> Dot Product/2, Subtract/2
  Gain/1 -> Product/2
  Product1/1 -> b_N/1
  Constant/1 -> Power/2
  Dot Product/1 -> Gain/1
  Subtract/1 -> Product1/2
  Norm of Vector H/1(Norm) -> Divide/1
  Power/1 -> Divide/2
  H0 vector/1 -> Norm of Vector H/1(Vector)

== system prova/Dynamics e Kinematics/Attitude error GG ==
  w : Inport
  DCM_B/N : Inport  Port=2
  Clock : Clock
  Constant : Constant  Value=n_e
  Constant5 : Constant  Value=0
  Matrix Multiply1 : Product  Multiplication=Matrix(*)
  Product : Product
  Subtract : Sum  Inputs=+-
  Vector Concatenate3 : Concatenate  NumInputs=3
  calculating A_B/L : Subsystem
  Ang Vel Error : Outport
  DCM_B/L : Outport  Port=2
  wires:
  Constant5/1 -> Vector Concatenate3/2, Vector Concatenate3/1
  Vector Concatenate3/1 -> Matrix Multiply1/2  "w_L/N"
  calculating A_B/L/1(A_B/L) -> Matrix Multiply1/1, DCM_B/L/1
  Matrix Multiply1/1 -> Subtract/2  "A_B/L * w_L/N"
  w/1 -> Subtract/1
  Subtract/1 -> Ang Vel Error/1
  Product/1 -> calculating A_B/L/1(Theta)  "Theta"
  Clock/1 -> Product/2
  Constant/1 -> Product/1, Vector Concatenate3/3
  DCM_B/N/1 -> calculating A_B/L/2(A_B/N)

== system prova/Dynamics e Kinematics/DCM composition from quaternions 1 ==
  q(4x1) : Inport
  Cross product matrix composition : Subsystem
  Demux : Demux
  Dot Product : DotProduct  OutDataTypeStr=Inherit: Inherit via internal rule
  Gain : Gain  Gain=[1 0 0; 0 1 0; 0 0 1]
  Gain1 : Gain  Gain=2
  Gain2 : Gain  Gain=-2
  Mux : Mux  Inputs=3
  Product : Product  Multiplication=Matrix(*)
  Product1 : Product
  Square : Math  Operator=square
  Sum : Sum  Inputs=|-+
  Sum1 : Sum  Inputs=+++
  Transpose : Math  Operator=transpose
  DCM : Outport
  wires:
  Gain/1 -> Sum1/1
  Demux/1 -> Mux/1
  q(4x1)/1 -> Demux/1
  Demux/2 -> Mux/2
  Mux/1 -> Dot Product/2, Dot Product/1, Product/1, Cross product matrix composition/1(q_vect), Transpose/1  "q_vect"
  Demux/4 -> Gain2/1, Square/1  "q4"
  Demux/3 -> Mux/3
  Dot Product/1 -> Sum/1
  Sum/1 -> Gain/1
  Square/1 -> Sum/2
  Transpose/1 -> Product/2
  Product/1 -> Gain1/1
  Gain2/1 -> Product1/2
  Cross product matrix composition/1(q_vect cross) -> Product1/1  "omega_mat"
  Product1/1 -> Sum1/3
  Gain1/1 -> Sum1/2
  Sum1/1 -> DCM/1

== system prova/Dynamics e Kinematics/Kinematics quaternion2 ==
  omega : Inport
  q0 : Inport  Port=2
  Demux : Demux
  Divide : Product  Inputs=*/
  Gain1 : Gain  Gain=-1
  Gain2 : Gain  Gain=-1
  Gain3 : Gain  Gain=1/2
  Gain4 : Gain  Gain=-1
  Integrator : Integrator  InitialConditionSource=external
  Matrix Multiply : Product  Multiplication=Matrix(*)
  Matrix OMEGA : Subsystem
  Mux : Mux
  Normalize Vector2 : Subsystem
  q : Outport
  q^(-1) : Outport  Port=2
  wires:
  Gain3/1 -> Matrix Multiply/1
  Matrix Multiply/1 -> Integrator/1
  omega/1 -> Matrix OMEGA/1(omega)
  Integrator/1 -> Normalize Vector2/1(Vector), Divide/1, Demux/1, q/1
  Matrix OMEGA/1(Matrix Omega) -> Gain3/1
  q0/1 -> Integrator/2
  Demux/2 -> Gain1/1
  Demux/3 -> Gain2/1
  Demux/4 -> Gain4/1
  Gain1/1 -> Mux/2
  Gain2/1 -> Mux/3
  Gain4/1 -> Mux/4
  Demux/1 -> Mux/1
  Mux/1 -> q^(-1)/1
  Normalize Vector2/1(Norm) -> Divide/2
  Divide/1 -> Matrix Multiply/2

== system prova/Dynamics e Kinematics/Single spin dynamics ==
  Inertia matrix inverse : Inport
  Inertia matrix : Inport  Port=2
  Omega_0 : Inport  Port=3
  M : Inport  Port=4
  Cross Product : matrix_library/Cross Product
  Integrator1 : Integrator  InitialConditionSource=external
  Product : Product  Multiplication=Matrix(*)
  Product1 : Product  Multiplication=Matrix(*)
  Scope2 : Scope
  Sum : Sum  Inputs=|++
  Transpose1 : Math  Operator=transpose
  Omega : Outport
  wires:
  Transpose1/1 -> Omega/1
  Inertia matrix inverse/1 -> Product/1
  Integrator1/1 -> Product1/2, Transpose1/1, Cross Product/2, Scope2/1  "omega"
  Product/1 -> Integrator1/1  "omega_dot"
  Omega_0/1 -> Integrator1/2
  Product1/1 -> Cross Product/1
  Inertia matrix/1 -> Product1/1
  Cross Product/1 -> Sum/1
  Sum/1 -> Product/2
  M/1 -> Sum/2

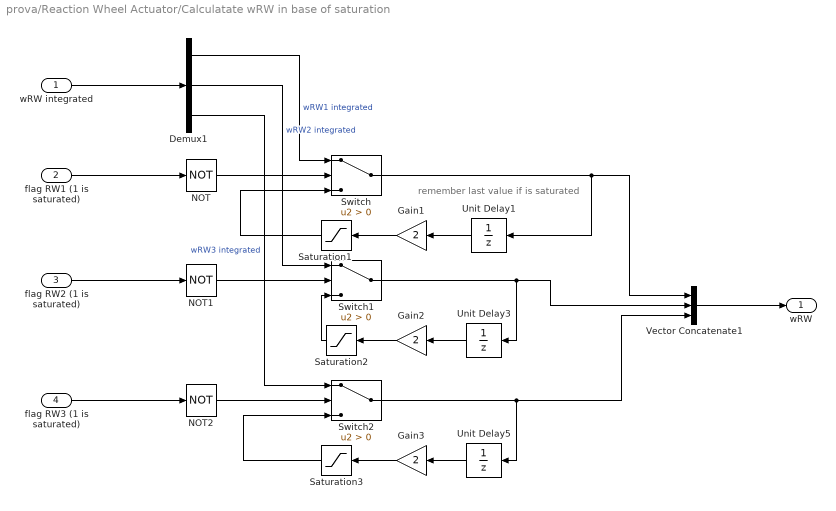
== system prova/Reaction Wheel Actuator/Calculatate wRW in base of saturation ==
  note: remember last value if is saturated
  wRW integrated : Inport
  flag RW1 (1 is saturated) : Inport  Port=2
  flag RW2 (1 is saturated) : Inport  Port=3
  flag RW3 (1 is saturated) : Inport  Port=4
  Demux1 : Demux  Outputs=3
  Gain1 : Gain  Gain=2
  Gain2 : Gain  Gain=2
  Gain3 : Gain  Gain=2
  NOT : Logic  Operator=NOT  IconShape=distinctive  AllPortsSameDT=off  OutDataTypeStr=boolean
  NOT1 : Logic  Operator=NOT  IconShape=distinctive  AllPortsSameDT=off  OutDataTypeStr=boolean
  NOT2 : Logic  Operator=NOT  IconShape=distinctive  AllPortsSameDT=off  OutDataTypeStr=boolean
  Saturation1 : Saturate  UpperLimit=wMax_RW  LowerLimit=-wMax_RW
  Saturation2 : Saturate  UpperLimit=wMax_RW  LowerLimit=-wMax_RW
  Saturation3 : Saturate  UpperLimit=wMax_RW  LowerLimit=-wMax_RW
  Switch : Switch  Criteria=u2 > Threshold  SaturateOnIntegerOverflow=off  InputSameDT=off
  Switch1 : Switch  Criteria=u2 > Threshold  SaturateOnIntegerOverflow=off  InputSameDT=off
  Switch2 : Switch  Criteria=u2 > Threshold  SaturateOnIntegerOverflow=off  InputSameDT=off
  Unit Delay1 : UnitDelay  SampleTime=-1  HasFrameUpgradeWarning=on
  Unit Delay3 : UnitDelay  SampleTime=-1  HasFrameUpgradeWarning=on
  Unit Delay5 : UnitDelay  SampleTime=-1  HasFrameUpgradeWarning=on
  Vector Concatenate1 : Concatenate  NumInputs=3
  wRW : Outport
  wires:
  Gain2/1 -> Saturation2/1
  Switch1/1 -> Unit Delay3/1, Vector Concatenate1/2
  NOT/1 -> Switch/2
  flag RW1 (1 is saturated)/1 -> NOT/1
  Saturation3/1 -> Switch2/3
  NOT1/1 -> Switch1/2
  Saturation2/1 -> Switch1/3
  wRW integrated/1 -> Demux1/1
  Switch2/1 -> Unit Delay5/1, Vector Concatenate1/3
  Unit Delay5/1 -> Gain3/1
  Unit Delay3/1 -> Gain2/1
  Demux1/2 -> Switch1/1  "wRW2 integrated"
  Gain1/1 -> Saturation1/1
  Vector Concatenate1/1 -> wRW/1
  Switch/1 -> Unit Delay1/1, Vector Concatenate1/1
  Unit Delay1/1 -> Gain1/1
  Saturation1/1 -> Switch/3
  Demux1/3 -> Switch2/1  "wRW3 integrated"
  Demux1/1 -> Switch/1  "wRW1 integrated"
  NOT2/1 -> Switch2/2
  Gain3/1 -> Saturation3/1
  flag RW3 (1 is saturated)/1 -> NOT2/1
  flag RW2 (1 is saturated)/1 -> NOT1/1

== system prova/Reaction Wheel Actuator/Subsystem1 ==
  h_r dot : Inport
  flag RW1 (1 is saturated) : Inport  Port=2
  flag RW2 (1 is saturated) : Inport  Port=3
  flag RW3 (1 is saturated) : Inport  Port=4
  Constant10 : Constant  Value=0
  Constant11 : Constant  Value=0
  Constant7 : Constant  Value=0
  Demux3 : Demux  Outputs=3
  Switch1 : Switch  Criteria=u2 > Threshold  SaturateOnIntegerOverflow=off  InputSameDT=off
  Switch2 : Switch  Criteria=u2 > Threshold  SaturateOnIntegerOverflow=off  InputSameDT=off
  Switch3 : Switch  Criteria=u2 > Threshold  SaturateOnIntegerOverflow=off  InputSameDT=off
  Vector Concatenate2 : Concatenate  NumInputs=3
  M : Outport
  wires:
  Demux3/3 -> Switch2/3
  Constant11/1 -> Switch2/1
  Switch2/1 -> Vector Concatenate2/3
  Demux3/1 -> Switch3/3
  Demux3/2 -> Switch1/3
  Switch3/1 -> Vector Concatenate2/1
  Switch1/1 -> Vector Concatenate2/2
  flag RW3 (1 is saturated)/1 -> Switch2/2
  Constant7/1 -> Switch3/1
  Constant10/1 -> Switch1/1
  flag RW1 (1 is saturated)/1 -> Switch3/2
  h_r dot/1 -> Demux3/1
  flag RW2 (1 is saturated)/1 -> Switch1/2
  Vector Concatenate2/1 -> M/1

== system prova/Reaction Wheel Actuator/detect if the RW is saturated (output == 1 isSaturated) ==
  w : Inport
  Abs : Abs  SaturateOnIntegerOverflow=off
  Compare To Constant : simulink/Logic and Bit Operations/Compare To Constant  relop=>=  const=wMax_RW  OutDataTypeStr=boolean
  Demux : Demux  Outputs=3
  Logical Operator : Logic  Operator=OR  AllPortsSameDT=off  OutDataTypeStr=boolean
  Logical Operator1 : Logic  Operator=OR  AllPortsSameDT=off  OutDataTypeStr=boolean
  Logical Operator2 : Logic  Operator=OR  AllPortsSameDT=off  OutDataTypeStr=boolean
  Unit Delay : UnitDelay  SampleTime=-1  HasFrameUpgradeWarning=on
  Unit Delay2 : UnitDelay  SampleTime=-1  HasFrameUpgradeWarning=on
  Unit Delay4 : UnitDelay  SampleTime=-1  HasFrameUpgradeWarning=on
  flag RW1 : Outport
  flag RW2 : Outport  Port=2
  flag RW3 : Outport  Port=3
  wires:
  Unit Delay4/1 -> Logical Operator2/2
  Unit Delay/1 -> Logical Operator/2
  Demux/1 -> Logical Operator/1
  Logical Operator/1 -> flag RW1/1, Unit Delay/1
  Unit Delay2/1 -> Logical Operator1/2
  Logical Operator2/1 -> flag RW3/1, Unit Delay4/1
  Demux/2 -> Logical Operator1/1
  Logical Operator1/1 -> flag RW2/1, Unit Delay2/1
  Demux/3 -> Logical Operator2/1
  Abs/1 -> Compare To Constant/1
  w/1 -> Abs/1
  Compare To Constant/1 -> Demux/1

== system prova/Statistical methods attitude determination (quaternion  Wabha’s problem) /For Iterator Subsystem to calculate B matrix ==
  note: Remember the last matrix B
  note: count the index
      | Important to flag reset in "State variable" to reset unit delay
  note: It's a for loop that resolve this expression
      | 𝐵 = ∑ 𝛼_𝑖*𝑠_𝑖*𝑣_𝑖' = [𝑏ij] to obatain matix B that it is a square matrix of order 3
      |
      | Analogous code for the iteration:
      |
      | for i = 1:size(alpha,2)
      | B = B + alpha(i)*s(:,i)*v(:,i)'
      | end
  alpha : Inport
  s matrix : Inport  Port=2
  v matrix : Inport  Port=3
  Add : Sum
  For Iterator : ForIterator  ResetStates=reset  IterationLimit=size(alpha,2)
  Matrix Multiply : Product  Multiplication=Matrix(*)
  Product : Product
  Transpose : Math  Operator=transpose
  Unit Delay1 : UnitDelay  SampleTime=-1  HasFrameUpgradeWarning=on
  Variable Selector : dspindex/Variable Selector  NumInputs=1  rowsOrCols=Columns  IdxMode=Variable  Elements=[1 3]  ZerOneIdxMode=One-based  errmode=Clip Index  FillMode=on  FillValues=0
  Variable Selector1 : dspindex/Variable Selector  NumInputs=1  rowsOrCols=Columns  IdxMode=Variable  Elements=[1 3]  ZerOneIdxMode=One-based  errmode=Clip Index  FillMode=on  FillValues=0
  Variable Selector2 : dspindex/Variable Selector  NumInputs=1  rowsOrCols=Columns  IdxMode=Variable  Elements=[1 3]  ZerOneIdxMode=One-based  errmode=Clip Index  FillMode=on  FillValues=0
  B matrix : Outport
  wires:
  For Iterator/1 -> Variable Selector1/2, Variable Selector/2, Variable Selector2/2
  alpha/1 -> Variable Selector2/1
  s matrix/1 -> Variable Selector/1
  Variable Selector2/1 -> Product/1
  Variable Selector/1 -> Product/2
  Product/1 -> Matrix Multiply/1
  Variable Selector1/1 -> Transpose/1
  Transpose/1 -> Matrix Multiply/2
  Matrix Multiply/1 -> Add/1
  v matrix/1 -> Variable Selector1/1
  Unit Delay1/1 -> Add/2
  Add/1 -> Unit Delay1/1, B matrix/1

== system prova/Statistical methods attitude determination (quaternion  Wabha’s problem) /Matrix trace ==
  Matrix : Inport
  Extract Diagonal : matrix_library/Extract Diagonal
      settings: LibrarySourceBlock=|
      | simulink/Matrix
      | Operations/Extract Diagonal
  Sum of Elements : Sum  Inputs=+
  trace : Outport
  wires:
  Extract Diagonal/1 -> Sum of Elements/1
  Sum of Elements/1 -> trace/1  "sigma"
  Matrix/1 -> Extract Diagonal/1

== system prova/Statistical methods attitude determination (quaternion  Wabha’s problem) /Vector z ==
  B : Inport
  Gain1 : Gain  Gain=-1
  Selector : Selector  NumberOfDimensions=2  InputPortWidth=3  IndexOptions=Index vector (dialog),Starting index (dialog)  Indices=2,3  OutputSizes=1,1
  Selector1 : Selector  NumberOfDimensions=2  InputPortWidth=3  IndexOptions=Index vector (dialog),Starting index (dialog)  Indices=1,3  OutputSizes=1,1
  Selector2 : Selector  NumberOfDimensions=2  InputPortWidth=3  IndexOptions=Index vector (dialog),Starting index (dialog)  Indices=1,2  OutputSizes=1,1
  Subtract1 : Sum  Inputs=+-
  Transpose1 : Math  Operator=transpose
  Vector Concatenate : Concatenate  NumInputs=3
  z : Outport
  wires:
  B/1 -> Subtract1/1, Transpose1/1
  Transpose1/1 -> Subtract1/2
  Selector2/1 -> Vector Concatenate/3
  Selector/1 -> Vector Concatenate/1
  Subtract1/1 -> Selector/1, Selector2/1, Selector1/1
  Vector Concatenate/1 -> z/1
  Gain1/1 -> Vector Concatenate/2
  Selector1/1 -> Gain1/1

== system prova/Subsystem/DCM to quaternion ==
  DCM : Inport
  Constant : Constant
  Divide : Product  Inputs=*/
  Extract Diagonal : matrix_library/Extract Diagonal
      settings: LibrarySourceBlock=|
      | simulink/Matrix
      | Operations/Extract Diagonal
  Gain : Gain  Gain=0.5
  Gain1 : Gain  Gain=[0 0 0; 0 0 1; 0 -1 0]
  Gain2 : Gain  Gain=[0 0 -1; 0 0 0; 1 0 0]
  Gain3 : Gain  Gain=[0 1 0; -1 0 0; 0 0 0]
  Gain4 : Gain  Gain=4
  Normalize Vector1 : Subsystem
  Sqrt : Sqrt
  Sum : Sum  Inputs=|++
  Sum of Elements{,1..3} (4 alike) : Sum  Inputs=+
  Vector Concatenate : Concatenate  NumInputs=3
  Vector Concatenate1 : Concatenate
  q (scalar last) : Outport
  wires:
  Extract Diagonal/1 -> Sum of Elements/1
  Sum of Elements/1 -> Sum/1
  Constant/1 -> Sum/2
  Sum/1 -> Sqrt/1
  Sqrt/1 -> Gain/1
  DCM/1 -> Gain1/1, Gain2/1, Gain3/1, Extract Diagonal/1
  Gain2/1 -> Sum of Elements1/1
  Sum of Elements1/1 -> Vector Concatenate/2
  Gain1/1 -> Sum of Elements2/1
  Sum of Elements2/1 -> Vector Concatenate/1
  Sum of Elements3/1 -> Vector Concatenate/3
  Gain3/1 -> Sum of Elements3/1
  Vector Concatenate/1 -> Divide/1
  Gain/1 -> Vector Concatenate1/2, Gain4/1
  Gain4/1 -> Divide/2
  Divide/1 -> Vector Concatenate1/1
  Vector Concatenate1/1 -> Normalize Vector1/1(Vector)
  Normalize Vector1/1(Versor) -> q (scalar last)/1

== system prova/Subsystem/Norm vector ==
  Vector : Inport
  Dot Product : DotProduct  OutDataTypeStr=Inherit: Inherit via internal rule
  Sqrt : Sqrt
  Norm : Outport
  wires:
  Sqrt/1 -> Norm/1
  Vector/1 -> Dot Product/1, Dot Product/2
  Dot Product/1 -> Sqrt/1

== system prova/Subsystem/Normalize Vector1 ==
  Vector : Inport
  Divide : Product  Inputs=*/
  Norm vector : Subsystem  AncestorBlock=LibrarySAD5/Normalize Vector1
  Versor : Outport
  wires:
  Vector/1 -> Norm vector/1(Vector), Divide/1
  Divide/1 -> Versor/1
  Norm vector/1(Norm) -> Divide/2

== system prova/Subsystem/Normalize Vector2 ==
  Vector : Inport
  Divide : Product  Inputs=*/
  Norm vector : Subsystem  AncestorBlock=LibrarySAD5/Normalize Vector1
  Versor : Outport
  wires:
  Vector/1 -> Norm vector/1(Vector), Divide/1
  Divide/1 -> Versor/1
  Norm vector/1(Norm) -> Divide/2

== system prova/Subsystem/Normalize Vector3 ==
  Vector : Inport
  Divide : Product  Inputs=*/
  Norm vector : Subsystem  AncestorBlock=LibrarySAD5/Normalize Vector1
  Versor : Outport
  wires:
  Vector/1 -> Norm vector/1(Vector), Divide/1
  Divide/1 -> Versor/1
  Norm vector/1(Norm) -> Divide/2

== system prova/Subsystem/Normalize Vector4 ==
  Vector : Inport
  Divide : Product  Inputs=*/
  Norm vector : Subsystem  AncestorBlock=LibrarySAD5/Normalize Vector1
  Versor : Outport
  wires:
  Vector/1 -> Norm vector/1(Vector), Divide/1
  Divide/1 -> Versor/1
  Norm vector/1(Norm) -> Divide/2

== system prova/Subsystem1/Normalize Vector1 ==
  Vector : Inport
  Divide : Product  Inputs=*/
  Norm vector : Subsystem  AncestorBlock=LibrarySAD5/Normalize Vector1
  Versor : Outport
  wires:
  Vector/1 -> Norm vector/1(Vector), Divide/1
  Divide/1 -> Versor/1
  Norm vector/1(Norm) -> Divide/2

== system prova/Sun sensor (Da fare sistmando vettore e eclissi)/Normalize Vector1 ==
  Vector : Inport
  Divide : Product  Inputs=*/
  Normalize Vector : Subsystem  AncestorBlock=LibrarySAD5/Normalize Vector1
  Versor : Outport
  wires:
  Vector/1 -> Normalize Vector/1(Vector), Divide/1
  Divide/1 -> Versor/1
  Normalize Vector/1(Norm) -> Divide/2

== system prova/TRIAD: Attitude determination algebric Method with 2 sensor/Normalize Vector1 ==
  Vector : Inport
  Divide : Product  Inputs=*/
  Normalize Vector : Subsystem  AncestorBlock=LibrarySAD5/Normalize Vector1
  Versor : Outport
  wires:
  Vector/1 -> Normalize Vector/1(Vector), Divide/1
  Divide/1 -> Versor/1
  Normalize Vector/1(Norm) -> Divide/2

== system prova/TRIAD: Attitude determination algebric Method with 2 sensor/Normalize Vector2 ==
  Vector : Inport
  Divide : Product  Inputs=*/
  Norm vector : Subsystem  AncestorBlock=LibrarySAD5/Normalize Vector1
  Versor : Outport
  wires:
  Vector/1 -> Norm vector/1(Vector), Divide/1
  Divide/1 -> Versor/1
  Norm vector/1(Norm) -> Divide/2

== system prova/TRIAD: Attitude determination algebric Method with 2 sensor/Normalize Vector3 ==
  Vector : Inport
  Divide : Product  Inputs=*/
  Normalize Vector : Subsystem  AncestorBlock=LibrarySAD5/Normalize Vector1
  Versor : Outport
  wires:
  Vector/1 -> Normalize Vector/1(Vector), Divide/1
  Divide/1 -> Versor/1
  Normalize Vector/1(Norm) -> Divide/2
